simulink model "smith_pre"  (R2020b)
settings: Solver=VariableStepAuto  StartTime=0.0  StopTime=20  RelTol=1e-3
values from neighbouring files (symbols this model uses):
  delay1 = 2    [smith_pre_m.m]
  delay2 = 2.5    [smith_pre_m.m]
  K1 = 1    [smith_pre_m.m]
  K2 = 1.5    [smith_pre_m.m]
  T1 = 2    [smith_pre_m.m]
  T2 = 2.5    [smith_pre_m.m]
settings Model: Creator=huang  LastModifiedBy=huang

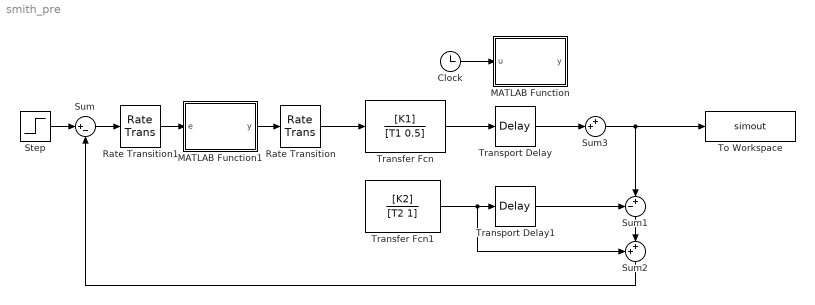
== system smith_pre ==
  Clock : Clock
  MATLAB Function : MATLAB Function  TreatAsAtomicUnit=on
  MATLAB Function1 : MATLAB Function  TreatAsAtomicUnit=on
  Rate Transition : RateTransition
  Rate Transition1 : RateTransition  OutPortSampleTime=5
  Step : Step  Time=0  SampleTime=0
  Sum : Sum  Inputs=|+-
  Sum1 : Sum  Inputs=-+|
  Sum2 : Sum  Inputs=++|
  Sum3 : Sum  Inputs=++|
  To Workspace : ToWorkspace  VariableName=simout  SampleTime=-1
      settings: Save2DSignal=2-D array (concatenate along first dimension)
  Transfer Fcn : TransferFcn  Numerator=[K1]  Denominator=[T1 0.5]
  Transfer Fcn1 : TransferFcn  Numerator=[K2]  Denominator=[T2 1]
  Transport Delay : TransportDelay  DelayTime=delay1
  Transport Delay1 : TransportDelay  DelayTime=delay2
  wires:
  Transfer Fcn/1 -> Transport Delay/1
  Step/1 -> Sum/1
  Transport Delay1/1 -> Sum1/1
  Sum1/1 -> Sum2/2
  Transfer Fcn1/1 -> Sum2/1, Transport Delay1/1
  Sum2/1 -> Sum/2
  Clock/1 -> MATLAB Function/1(u)
  Transport Delay/1 -> Sum3/2
  Sum3/1 -> Sum1/2, To Workspace/1
  MATLAB Function1/1(y) -> Rate Transition/1
  Rate Transition1/1 -> MATLAB Function1/1(e)
  Rate Transition/1 -> Transfer Fcn/1
  Sum/1 -> Rate Transition1/1

== matlab function smith_pre/MATLAB Function ==
  data: u input; y output
function y = fcn(u)
if(u<=5&&u>=4)
    y=-0.2;
else
    y=0;
end

== matlab function smith_pre/MATLAB Function1 ==
  data: e input; y output
function y = fcn(e)

y = e;
